simulink subsystem "PvtSubSys_VSM_LKA"  (R2020b)
settings: Solver=VariableStepAuto  StartTime=0.0  StopTime=10.0  RelTol=1e-3
values from neighbouring files (symbols this model uses):
  P_VSM_LKA_AbsEspInTime = 3.0    [LKA.sldd]
  P_VSM_LKA_absLongitudeAcceIn = 2.5    [LKA.sldd]
  P_VSM_LKA_absLongitudeAcceInTime = 3.0    [LKA.sldd]
  P_VSM_LKA_absLongitudeAcceOut = 3.0    [LKA.sldd]
  P_VSM_LKA_AccPedalPosnOut = 30.0    [LKA.sldd]
  P_VSM_LKA_AccPedalRateOutTime = 0.0    [LKA.sldd]
  P_VSM_LKA_AccRateIn = 30.0    [LKA.sldd]
  P_VSM_LKA_AccRateInTime = 1.5    [LKA.sldd]
  P_VSM_LKA_AccRateOut = 70.0    [LKA.sldd]
  P_VSM_LKA_BrakePressIn = 3.0    [LKA.sldd]
  P_VSM_LKA_BrakePressInTime = 1.5    [LKA.sldd]
  P_VSM_LKA_BrakePressOut = 5.0    [LKA.sldd]
  P_VSM_LKA_CurveFactor = 1.0    [LKA.sldd]
  P_VSM_LKA_DriverInputTrqValueIn = 2.0    [LKA.sldd]
  P_VSM_LKA_DriverInputTrqValueInTime = 3.0    [LKA.sldd]
  P_VSM_LKA_DriverInputTrqValueOut = 2.3    [LKA.sldd]
  P_VSM_LKA_EndSwitch = 1.0    [LKA.sldd]
  P_VSM_LKA_LaneChangeOffset = 0.11    [LKA.sldd]
  P_VSM_LKA_LaneCurveIn = 0.005    [LKA.sldd]
  P_VSM_LKA_LaneCurveOut = 0.006    [LKA.sldd]
  P_VSM_LKA_LateralAcceIn = 3.0    [LKA.sldd]
  P_VSM_LKA_LateralAcceInTime = 3.0    [LKA.sldd]
  P_VSM_LKA_LateralAcceOut = 3.5    [LKA.sldd]
  P_VSM_LKA_LongitudeAcceIn = 3.0    [LKA.sldd]
  P_VSM_LKA_LongitudeAcceOut = 3.5    [LKA.sldd]
  P_VSM_LKA_OverrideInTime = 1.5    [LKA.sldd]
  P_VSM_LKA_OverrideTime = 0.3    [LKA.sldd]
  P_VSM_LKA_OverrideValue = 1.2    [LKA.sldd]
  P_VSM_LKA_State_Absesp_enable = 1.0    [LKA.sldd]
  P_VSM_LKA_State_Accpedalrate_enable = 1.0    [LKA.sldd]
  P_VSM_LKA_State_Breakpressure_enable = 1.0    [LKA.sldd]
  P_VSM_LKA_State_DriverInputTrqValue_enable = 1.0    [LKA.sldd]
  P_VSM_LKA_State_Eps_enable = 1.0    [LKA.sldd]
  P_VSM_LKA_State_ESSSts_enable = 1.0    [LKA.sldd]
  P_VSM_LKA_State_Failsafe_enable = 1.0    [LKA.sldd]
  P_VSM_LKA_State_GEAR_enable = 1.0    [LKA.sldd]
  P_VSM_LKA_State_Handson_enable = 1.0    [LKA.sldd]
  P_VSM_LKA_State_Headingangle_enable = 1.0    [LKA.sldd]
  P_VSM_LKA_State_Lane_enable = 1.0    [LKA.sldd]
  P_VSM_LKA_State_LaneChange_enable = 1.0    [LKA.sldd]
  P_VSM_LKA_State_Lanecurve_enable = 1.0    [LKA.sldd]
  P_VSM_LKA_State_LateralAcce_enable = 1.0    [LKA.sldd]
  P_VSM_LKA_State_LongitudeAcc_enable = 1.0    [LKA.sldd]
  P_VSM_LKA_State_Overide_enable = 1.0    [LKA.sldd]
  P_VSM_LKA_State_Param_AngleOffset = 0.15    [LKA.sldd]
  P_VSM_LKA_State_Param_InterventionZoneIn = 0.4    [LKA.sldd]
  P_VSM_LKA_State_Param_InterventionZoneOut = -0.65    [LKA.sldd]
  P_VSM_LKA_State_Param_LaneCurve : value not decoded    [LKA.sldd]
  P_VSM_LKA_State_Param_LaneCurve_Offset : value not decoded    [LKA.sldd]
  P_VSM_LKA_State_Param_LaneWidth_Offset : value not decoded    [LKA.sldd]
  P_VSM_LKA_State_Param_OutOffset = 0.2    [LKA.sldd]
  P_VSM_LKA_State_Param_REInterventionZoneIn = 0.55    [LKA.sldd]
  P_VSM_LKA_State_Param_Sensitive_Offset : value not decoded    [LKA.sldd]
  P_VSM_LKA_State_SteerWheelAngle_enable = 1.0    [LKA.sldd]
  P_VSM_LKA_State_SteerWheelSpd_enable = 1.0    [LKA.sldd]
  P_VSM_LKA_State_TJASts_enable = 1.0    [LKA.sldd]
  P_VSM_LKA_State_TurnLight_enable = 1.0    [LKA.sldd]
  P_VSM_LKA_State_Vehspeed_enable = 1.0    [LKA.sldd]
  P_VSM_LKA_State_Yawsup_enable = 1.0    [LKA.sldd]
  P_VSM_LKA_SteerWheelAngleIn = 70.0    [LKA.sldd]
  P_VSM_LKA_SteerWheelAngleInTime = 3.0    [LKA.sldd]
  P_VSM_LKA_SteerWheelAngleOut = 90.0    [LKA.sldd]
  P_VSM_LKA_SteerWheelSpdIn = 150.0    [LKA.sldd]
  P_VSM_LKA_SteerWheelSpdInTime = 3.0    [LKA.sldd]
  P_VSM_LKA_SteerWheelSpdOut = 200.0    [LKA.sldd]
  P_VSM_LKA_TurnLightInTime = 3.0    [LKA.sldd]
  P_VSM_LKA_Warnarea1 = -0.55    [LKA.sldd]
  P_VSM_LKA_Warnarea2 = -0.35    [LKA.sldd]
  P_VSM_LKA_WarnInTime = 2.0    [LKA.sldd]
  P_VSM_LKA_WhelDy = 2.0    [LKA.sldd]
  P_VSM_LKA_YawRateIn = 0.2    [LKA.sldd]
  P_VSM_LKA_YawRateInTime = 1.0    [LKA.sldd]
  P_VSM_LKA_YawRateOut = 0.25    [LKA.sldd]
undefined symbols (not defined in the file or in its folder): P_VSM_LKA_AddOffset, P_VSM_LSMC_SampleTime, STATE
libraries: simulink x162
(part 5 of 5)

== matlab function PvtSubSys_VSM_LKA/LKA2/LKA/MATLAB Function1 ==
  data: active_fg input boolean size=1; PreFLWhelDy input single size=1; PreFRWhelDy input single size=1; FLWhelDy input single size=1; FRWhelDy input single size=1; Left_Valid input boolean size=1; Right_Valid input boolean size=1; OutOffset input single size=1; LKA_active output single size=1; LKA_Out output single size=1; LKA_End output single size=1; ReactionZoneInDy_m input double size=1; ReactionZoneOutDy_m input single size=1; Angleoffset input single size=1; TargetLine input single size=1; HeadingAngel input single size=1; lfgk1 input single size=1; lfg output single size=1; loutk1 input single size=1; lout output single size=1; rfgk1 input single size=1; routk1 input single size=1; rfg output single size=1; rout output single size=1
function [LKA_active,LKA_Out,LKA_End,lfg,lout,rfg,rout]  = fcn(active_fg,PreFLWhelDy,PreFRWhelDy,FLWhelDy,FRWhelDy,......
    Left_Valid,Right_Valid,OutOffset,ReactionZoneInDy_m,ReactionZoneOutDy_m,Angleoffset,TargetLine,HeadingAngel,lfgk1,loutk1,rfgk1,routk1)

LKA_active=single(0);
LKA_Out=single(0);
LKA_End=single(0);
lfg=single(0);
rfg=single(0);
lout=single(0);
rout=single(0);
if Left_Valid>0 && active_fg==single(1) 
    if  PreFLWhelDy<ReactionZoneInDy_m && PreFLWhelDy>ReactionZoneOutDy_m % 进入区域 -0.9--0.4
        if loutk1==single(1)
            lout=single(1);
            LKA_End=single(0);
            lfg=single(0);
        else
            LKA_active= single(1);
            lfg=single(1);
            lout=single(0);
        end
    elseif TargetLine<-OutOffset  &&  FLWhelDy>ReactionZoneOutDy_m && lfgk1>0 %扩大
        if loutk1==single(1)
            lout=single(1);
            LKA_End=single(0);
            lfg=single(0);
        else
            LKA_active= single(1);
            lfg=single(1);
            lout=single(0);
        end
    elseif TargetLine>-OutOffset && TargetLine<OutOffset && HeadingAngel>-Angleoffset && HeadingAngel< Angleoffset%稳定保持退出
        if loutk1==single(1)
            lout=single(1);
            LKA_End=single(0);
            lfg=single(0);
        else
            lfg=single(0);
            lout=single(0);
            LKA_Out=single(1);
        end

         
    elseif FLWhelDy < ReactionZoneOutDy_m   % 驶出 -0.9m
        lout=single(1);
        LKA_End=single(1);
    elseif FLWhelDy > ReactionZoneInDy_m + 0.1  
        lout=single(0);
   
         
    end
end

if Right_Valid>single(0) && active_fg==single(1)
    if  PreFRWhelDy<ReactionZoneInDy_m && PreFRWhelDy>ReactionZoneOutDy_m % 进入区域
        if routk1==single(1)
            rout=single(1);
            LKA_End=single(0);
            rfg=single(0);
        else
            LKA_active= single(2);
            rfg=single(1);
            rout=single(0);
        end
    elseif TargetLine<-OutOffset  &&  FRWhelDy>ReactionZoneOutDy_m && rfgk1>0
        if routk1==single(1)
            rout=single(1);
            LKA_End=single(0);
            rfg=single(0);
        else
            LKA_active= single(2);
            rfg=single(1);
            rout=single(0);
        end
    elseif TargetLine>-OutOffset && TargetLine<OutOffset && HeadingAngel>-Angleoffset && HeadingAngel< Angleoffset
        if routk1==single(1)
            rout=single(1);
            LKA_End=single(0);
            rfg=single(0);
        else
            rfg=single(0);
            rout=single(0);
            LKA_Out=single(1);
        end

         
    elseif FRWhelDy < ReactionZoneOutDy_m   % 驶出 -0.9m
        rout=single(1);
        LKA_End=single(1);
    elseif FRWhelDy > ReactionZoneInDy_m+0.1
        rout=single(0);
    
        
    end
end

if Left_Valid==single(0) && Right_Valid==single(0)
    LKA_End=single(1);
end
